simulink model "Stc"  (Simulink 8.4)
settings: Solver=ode45  StartTime=0.0  StopTime=10.0  RelTol=1e-3
undefined symbols (not defined in the file): Normal, Stc_CatalyserHeatingDelay, Stc_EngSpdSetCatalyserHeating, Stc_EngSpdStartOverdrive, Stc_rpmEngSpedMax
settings Model: Creator=YAL9FE  LastModifiedBy=ric9fe
settings DebuggingCC: FcnCallInpInsideContextMsg=EnableAllAsWarning

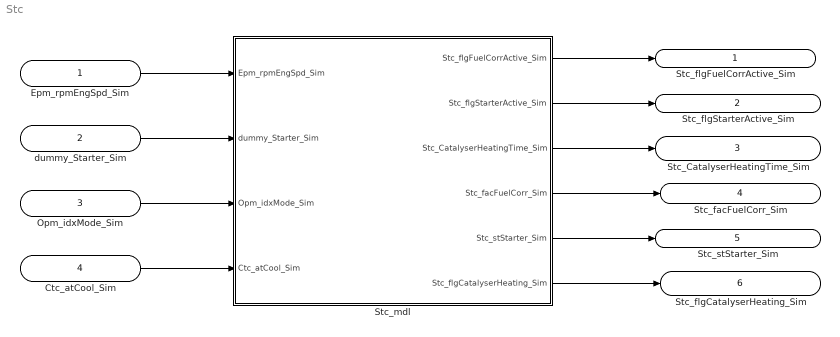
== system Stc ==
  Epm_rpmEngSpd_Sim : Inport
  dummy_Starter_Sim : Inport  Port=2
  Opm_idxMode_Sim : Inport  Port=3
  Ctc_atCool_Sim : Inport  Port=4
  Stc_mdl : Subsystem  mask(Functions){}
      mask help: StarterControl
      mask Display:
      | image(imread('StarterControl.jpg'))
      | port_label('input',1,'Epm_rpmEngSpd_Sim')
      | port_label('input',2,'dummy_Starter_Sim')
      | port_label('input',3,'Opm_idxMode_Sim')
      | port_label('input',4,'Ctc_atCool_Sim')
      | port_label('output',1,'Stc_flgFuelCorrActive_Sim')
      | port_label('output',2,'Stc_flgStarterActive_Sim')
      | port_label('output',3,'Stc_CatalyserHeatingTime_Sim')
      | port_label('output',4,'Stc_facFuelCorr_Sim')
      | port_label('output',5,'Stc_stStarter_Sim')
      | port_label('output',6,'Stc_flgCatalyserHeating_Sim')
  Stc_flgFuelCorrActive_Sim : Outport
  Stc_flgStarterActive_Sim : Outport  Port=2
  Stc_CatalyserHeatingTime_Sim : Outport  Port=3
  Stc_facFuelCorr_Sim : Outport  Port=4
  Stc_stStarter_Sim : Outport  Port=5
  Stc_flgCatalyserHeating_Sim : Outport  Port=6
  wires:
  Epm_rpmEngSpd_Sim/1 -> Stc_mdl/1(Epm_rpmEngSpd_Sim)
  dummy_Starter_Sim/1 -> Stc_mdl/2(dummy_Starter_Sim)
  Opm_idxMode_Sim/1 -> Stc_mdl/3(Opm_idxMode_Sim)
  Ctc_atCool_Sim/1 -> Stc_mdl/4(Ctc_atCool_Sim)
  Stc_mdl/1(Stc_flgFuelCorrActive_Sim) -> Stc_flgFuelCorrActive_Sim/1
  Stc_mdl/2(Stc_flgStarterActive_Sim) -> Stc_flgStarterActive_Sim/1
  Stc_mdl/3(Stc_CatalyserHeatingTime_Sim) -> Stc_CatalyserHeatingTime_Sim/1
  Stc_mdl/4(Stc_facFuelCorr_Sim) -> Stc_facFuelCorr_Sim/1
  Stc_mdl/5(Stc_stStarter_Sim) -> Stc_stStarter_Sim/1
  Stc_mdl/6(Stc_flgCatalyserHeating_Sim) -> Stc_flgCatalyserHeating_Sim/1

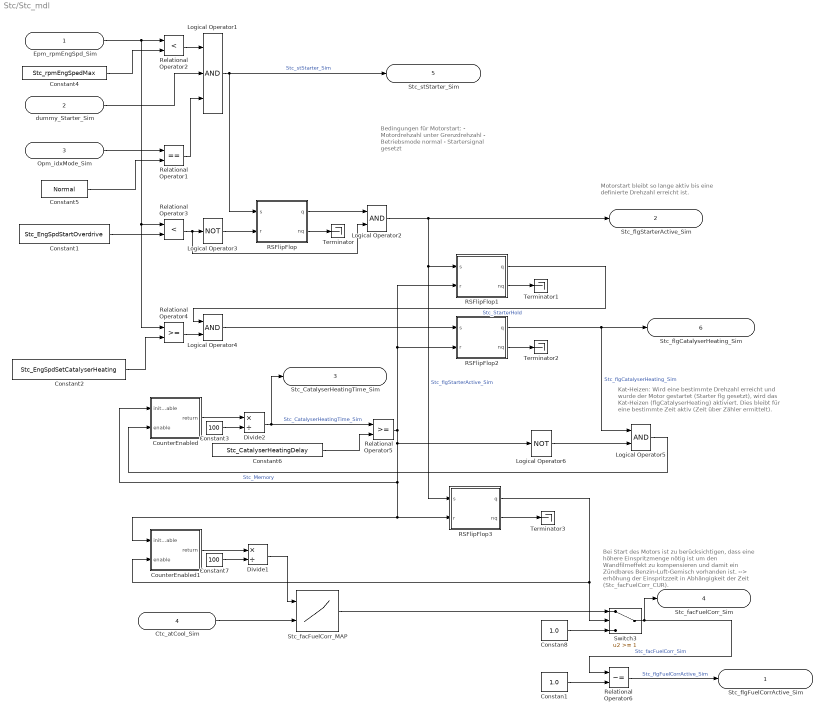
== system Stc/Stc_mdl ==
  note: Bedingungen für Motorstart:
      | - Motordrehzahl unter Grenzdrehzahl
      | - Betriebsmode normal
      | - Startersignal gesetzt
  note: Motorstart bleibt so lange aktiv bis
      | eine definierte Drehzahl erreicht ist.
  note: Kat-Heizen:
      | Wird eine bestimmte Drehzahl erreicht und wurde
      | der Motor gestartet (Starter flg gesetzt),
      | wird das Kat-Heizen (flgCatalyserHeating)
      | aktiviert. Dies bleibt für eine bestimmte Zeit aktiv
      | (Zeit über Zähler ermittelt).
  note: Bei Start des Motors ist zu berücksichtigen,
      | dass eine höhere Einspritzmenge nötig ist
      | um den Wandfilmeffekt zu kompensieren
      | und damit ein Zündbares Benzin-Luft-Gemisch
      | vorhanden ist.
      | --> erhöhung der Einspritzzeit in Abhängigkeit
      |       der Zeit (Stc_facFuelCorr_CUR).
  Epm_rpmEngSpd_Sim : Inport
  dummy_Starter_Sim : Inport  Port=2
  Opm_idxMode_Sim : Inport  Port=3
  Ctc_atCool_Sim : Inport  Port=4
  Constan1 : Constant  Value=1.0  OutDataTypeStr=single
  Constan8 : Constant  Value=1.0  OutDataTypeStr=single
  Constant1 : Constant  Value=Stc_EngSpdStartOverdrive
  Constant2 : Constant  Value=Stc_EngSpdSetCatalyserHeating
  Constant3 : Constant  Value=100  OutDataTypeStr=single
  Constant4 : Constant  Value=Stc_rpmEngSpedMax
  Constant5 : Constant  Value=Normal
  Constant6 : Constant  Value=Stc_CatalyserHeatingDelay
  Constant7 : Constant  Value=100  OutDataTypeStr=single
  CounterEnabled : Subsystem
      mask help: Counter
      mask Display: image(imread('CounterEnabled.jpg'))
  CounterEnabled1 : Subsystem
      mask help: Counter
      mask Display: image(imread('CounterEnabled.jpg'))
  Divide1 : Product  Inputs=*/  OutDataTypeStr=Inherit: Same as first input
  Divide2 : Product  Inputs=*/  OutDataTypeStr=Inherit: Same as first input
  Logical Operator1 : Logic  Inputs=3  AllPortsSameDT=off  OutDataTypeStr=boolean
  Logical Operator2 : Logic  AllPortsSameDT=off  OutDataTypeStr=boolean
  Logical Operator3 : Logic  Operator=NOT  AllPortsSameDT=off  OutDataTypeStr=boolean
  Logical Operator4 : Logic  AllPortsSameDT=off  OutDataTypeStr=boolean
  Logical Operator5 : Logic  AllPortsSameDT=off  OutDataTypeStr=boolean
  Logical Operator6 : Logic  Operator=NOT  AllPortsSameDT=off  OutDataTypeStr=boolean
  RSFlipFlop : Subsystem
      mask help: RSFlipFlop
      mask Display: image(imread('RSFlipFlop.jpg'))
  RSFlipFlop1 : Subsystem
      mask help: RSFlipFlop
      mask Display: image(imread('RSFlipFlop.jpg'))
  RSFlipFlop2 : Subsystem
      mask help: RSFlipFlop
      mask Display: image(imread('RSFlipFlop.jpg'))
  RSFlipFlop3 : Subsystem
      mask help: RSFlipFlop
      mask Display: image(imread('RSFlipFlop.jpg'))
  Relational Operator1 : RelationalOperator  Operator===  OutDataTypeStr=boolean
  Relational Operator2 : RelationalOperator  Operator=<  OutDataTypeStr=boolean
  Relational Operator3 : RelationalOperator  Operator=<  OutDataTypeStr=boolean
  Relational Operator4 : RelationalOperator  OutDataTypeStr=boolean
  Relational Operator5 : RelationalOperator  OutDataTypeStr=boolean
  Relational Operator6 : RelationalOperator  Operator=~=  OutDataTypeStr=boolean
  Stc_facFuelCorr_MAP : Lookup_n-D  BreakpointsForDimension1=[1:3]  BreakpointsForDimension2=[1:3]  ExtrapMethod=Clip  InputSameDT=on
  Switch3 : Switch  Threshold=1
  Terminator{,1..3} (4 alike) : Terminator
  Stc_flgFuelCorrActive_Sim : Outport
  Stc_flgStarterActive_Sim : Outport  Port=2
  Stc_CatalyserHeatingTime_Sim : Outport  Port=3
  Stc_facFuelCorr_Sim : Outport  Port=4
  Stc_stStarter_Sim : Outport  Port=5
  Stc_flgCatalyserHeating_Sim : Outport  Port=6
  wires:
  RSFlipFlop/2(nq) -> Terminator/1
  Epm_rpmEngSpd_Sim/1 -> Relational Operator2/1, Relational Operator3/1, Relational Operator4/1
  Relational Operator2/1 -> Logical Operator1/1
  Constant4/1 -> Relational Operator2/2
  dummy_Starter_Sim/1 -> Logical Operator1/2
  Opm_idxMode_Sim/1 -> Relational Operator1/1
  Constant5/1 -> Relational Operator1/2
  Relational Operator1/1 -> Logical Operator1/3
  Logical Operator1/1 -> Stc_stStarter_Sim/1, RSFlipFlop/1(s)  "Stc_stStarter_Sim"
  Constant1/1 -> Relational Operator3/2
  RSFlipFlop/1(q) -> Logical Operator2/1
  Relational Operator3/1 -> Logical Operator3/1, Logical Operator2/2
  Logical Operator3/1 -> RSFlipFlop/2(r)
  Logical Operator2/1 -> Stc_flgStarterActive_Sim/1, RSFlipFlop1/1(s), RSFlipFlop3/1(s)  "Stc_flgStarterActive_Sim"
  RSFlipFlop1/2(nq) -> Terminator1/1
  Constant2/1 -> Relational Operator4/2
  Relational Operator4/1 -> Logical Operator4/2
  RSFlipFlop1/1(q) -> Logical Operator4/1  "Stc_StarterHold"
  RSFlipFlop2/2(nq) -> Terminator2/1
  Logical Operator4/1 -> RSFlipFlop2/1(s)
  RSFlipFlop2/1(q) -> Stc_flgCatalyserHeating_Sim/1, Logical Operator5/1  "Stc_flgCatalyserHeating_Sim"
  CounterEnabled/1(return) -> Divide2/1
  Constant3/1 -> Divide2/2
  Divide2/1 -> Relational Operator5/1, Stc_CatalyserHeatingTime_Sim/1  "Stc_CatalyserHeatingTime_Sim"
  Constant6/1 -> Relational Operator5/2
  Relational Operator5/1 -> Logical Operator6/1, CounterEnabled/1(initEnable), CounterEnabled1/1(initEnable), RSFlipFlop3/2(r), RSFlipFlop2/2(r), RSFlipFlop1/2(r)  "Stc_Memory"
  Logical Operator6/1 -> Logical Operator5/2
  Logical Operator5/1 -> CounterEnabled/2(enable)
  RSFlipFlop3/2(nq) -> Terminator3/1
  CounterEnabled1/1(return) -> Divide1/1
  Constant7/1 -> Divide1/2
  RSFlipFlop3/1(q) -> CounterEnabled1/2(enable), Switch3/2
  Divide1/1 -> Stc_facFuelCorr_MAP/1
  Ctc_atCool_Sim/1 -> Stc_facFuelCorr_MAP/2
  Constan8/1 -> Switch3/3
  Stc_facFuelCorr_MAP/1 -> Switch3/1
  Switch3/1 -> Relational Operator6/1, Stc_facFuelCorr_Sim/1  "Stc_facFuelCorr_Sim"
  Relational Operator6/1 -> Stc_flgFuelCorrActive_Sim/1  "Stc_flgFuelCorrActive_Sim"
  Constan1/1 -> Relational Operator6/2

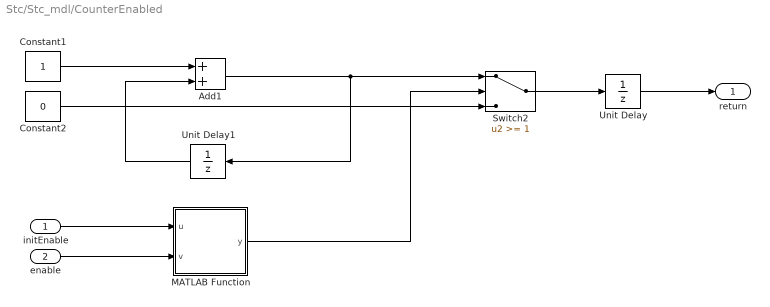
== system Stc/Stc_mdl/CounterEnabled ==
  initEnable : Inport
  enable : Inport  Port=2
  Add1 : Sum
  Constant1 : Constant  OutDataTypeStr=single
  Constant2 : Constant  Value=0  OutDataTypeStr=single
  MATLAB Function : MATLAB Function  TreatAsAtomicUnit=on
  Switch2 : Switch  Threshold=1
  Unit Delay : UnitDelay  SampleTime=-1
  Unit Delay1 : UnitDelay  SampleTime=-1
  return : Outport
  wires:
  initEnable/1 -> MATLAB Function/1(u)
  MATLAB Function/1(y) -> Switch2/2
  Add1/1 -> Unit Delay1/1, Switch2/1
  Constant2/1 -> Switch2/3
  Switch2/1 -> Unit Delay/1
  Unit Delay1/1 -> Add1/2
  Constant1/1 -> Add1/1
  enable/1 -> MATLAB Function/2(v)
  Unit Delay/1 -> return/1

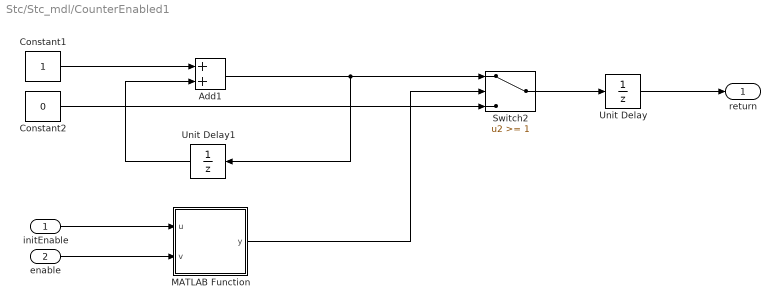
== system Stc/Stc_mdl/CounterEnabled1 ==
  initEnable : Inport
  enable : Inport  Port=2
  Add1 : Sum
  Constant1 : Constant  OutDataTypeStr=single
  Constant2 : Constant  Value=0  OutDataTypeStr=single
  MATLAB Function : MATLAB Function  TreatAsAtomicUnit=on
  Switch2 : Switch  Threshold=1
  Unit Delay : UnitDelay  SampleTime=-1
  Unit Delay1 : UnitDelay  SampleTime=-1
  return : Outport
  wires:
  enable/1 -> MATLAB Function/2(v)
  Constant1/1 -> Add1/1
  Unit Delay1/1 -> Add1/2
  Switch2/1 -> Unit Delay/1
  Constant2/1 -> Switch2/3
  Add1/1 -> Switch2/1, Unit Delay1/1
  MATLAB Function/1(y) -> Switch2/2
  initEnable/1 -> MATLAB Function/1(u)
  Unit Delay/1 -> return/1

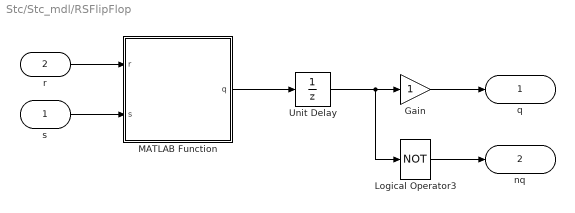
== system Stc/Stc_mdl/RSFlipFlop ==
  s : Inport
  r : Inport  Port=2
  Gain : Gain  OutDataTypeStr=Inherit: Same as input
  Logical Operator3 : Logic  Operator=NOT  AllPortsSameDT=off  OutDataTypeStr=boolean
  MATLAB Function : MATLAB Function  TreatAsAtomicUnit=on
  Unit Delay : UnitDelay  SampleTime=-1
  q : Outport
  nq : Outport  Port=2
  wires:
  MATLAB Function/1(q) -> Unit Delay/1
  s/1 -> MATLAB Function/2(s)
  r/1 -> MATLAB Function/1(r)
  Logical Operator3/1 -> nq/1
  Unit Delay/1 -> Logical Operator3/1, Gain/1
  Gain/1 -> q/1

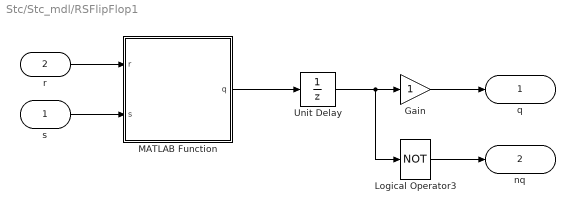
== system Stc/Stc_mdl/RSFlipFlop1 ==
  s : Inport
  r : Inport  Port=2
  Gain : Gain  OutDataTypeStr=Inherit: Same as input
  Logical Operator3 : Logic  Operator=NOT  AllPortsSameDT=off  OutDataTypeStr=boolean
  MATLAB Function : MATLAB Function  TreatAsAtomicUnit=on
  Unit Delay : UnitDelay  SampleTime=-1
  q : Outport
  nq : Outport  Port=2
  wires:
  Logical Operator3/1 -> nq/1
  r/1 -> MATLAB Function/1(r)
  s/1 -> MATLAB Function/2(s)
  MATLAB Function/1(q) -> Unit Delay/1
  Unit Delay/1 -> Logical Operator3/1, Gain/1
  Gain/1 -> q/1

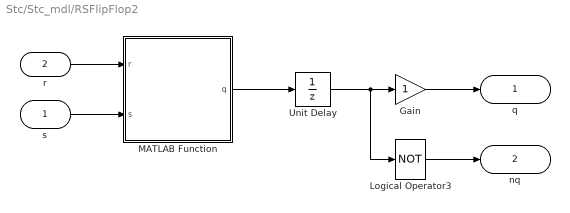
== system Stc/Stc_mdl/RSFlipFlop2 ==
  s : Inport
  r : Inport  Port=2
  Gain : Gain  OutDataTypeStr=Inherit: Same as input
  Logical Operator3 : Logic  Operator=NOT  AllPortsSameDT=off  OutDataTypeStr=boolean
  MATLAB Function : MATLAB Function  TreatAsAtomicUnit=on
  Unit Delay : UnitDelay  SampleTime=-1
  q : Outport
  nq : Outport  Port=2
  wires:
  MATLAB Function/1(q) -> Unit Delay/1
  s/1 -> MATLAB Function/2(s)
  r/1 -> MATLAB Function/1(r)
  Logical Operator3/1 -> nq/1
  Unit Delay/1 -> Logical Operator3/1, Gain/1
  Gain/1 -> q/1

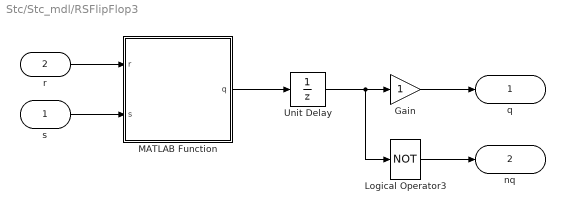
== system Stc/Stc_mdl/RSFlipFlop3 ==
  s : Inport
  r : Inport  Port=2
  Gain : Gain  OutDataTypeStr=Inherit: Same as input
  Logical Operator3 : Logic  Operator=NOT  AllPortsSameDT=off  OutDataTypeStr=boolean
  MATLAB Function : MATLAB Function  TreatAsAtomicUnit=on
  Unit Delay : UnitDelay  SampleTime=-1
  q : Outport
  nq : Outport  Port=2
  wires:
  Logical Operator3/1 -> nq/1
  r/1 -> MATLAB Function/1(r)
  s/1 -> MATLAB Function/2(s)
  MATLAB Function/1(q) -> Unit Delay/1
  Unit Delay/1 -> Logical Operator3/1, Gain/1
  Gain/1 -> q/1

== matlab function Stc_mdl/RSFlipFlop/MATLAB Function ==
  data: r input double; q output double; s input double
function q = fcn(r,s)
% FlipFlop
q = false;
if(r==true)
    q = false;
elseif(s==true)
    q = true;
end

== matlab function Stc_mdl/CounterEnabled/MATLAB Function ==
  data: u input double; y output double; v input double
function y = fcn(u,v)
% CounterEnabled Test
y = false;
if(u==true)
    y = false;
end
if(v==true)
    y = true;
end

== matlab function Stc_mdl/RSFlipFlop1/MATLAB Function ==
  data: r input double; q output double; s input double
function q = fcn(r,s)
% FlipFlop
q = false;
if(r==true)
    q = false;
elseif(s==true)
    q = true;
end

== matlab function Stc_mdl/RSFlipFlop2/MATLAB Function ==
  data: r input double; q output double; s input double
function q = fcn(r,s)
% FlipFlop
q = false;
if(r==true)
    q = false;
elseif(s==true)
    q = true;
end

== matlab function Stc_mdl/RSFlipFlop3/MATLAB Function ==
  data: r input double; q output double; s input double
function q = fcn(r,s)
% FlipFlop
q = false;
if(r==true)
    q = false;
elseif(s==true)
    q = true;
end

== matlab function Stc_mdl/CounterEnabled1/MATLAB Function ==
  data: u input double; y output double; v input double
function y = fcn(u,v)
% CounterEnabled Test
y = false;
if(u==true)
    y = false;
end
if(v==true)
    y = true;
end
